simulink model "TNN_model"  (R2024b)
settings: Solver=VariableStepAuto  StartTime=0.0  StopTime=stopTime  RelTol=1e-3
values from neighbouring files (symbols this model uses):
  initialCondition = squeeze(test_tensor(numInputs+1:end,:,1))    [TNN_matlab.m]
  modelParams = exportToSimulink(model)    [TNN_matlab.m]
  testID = 1    [TNN_matlab.m]
undefined symbols (not defined in the file or in its folder): extractdata
settings Model: Creator=cstockha  LastModifiedBy=cstockha
settings DebuggingCC: UnderspecifiedInitializationDetection=Classic  MergeDetectMultiDrivingBlocksExec=none
settings ModelReferenceCC: PropagateSignalLabelsOutOfModel=off

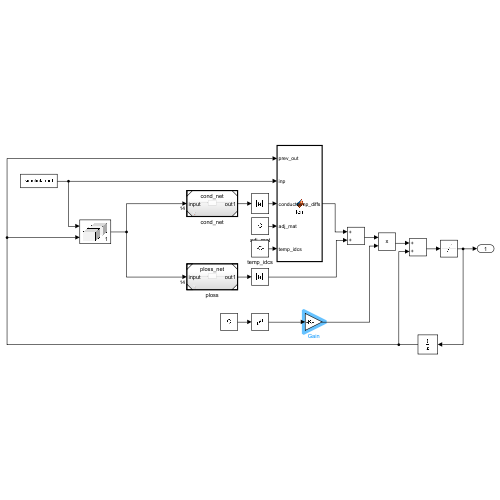
[thumbnail: Simulink's stored preview of the top-level diagram]
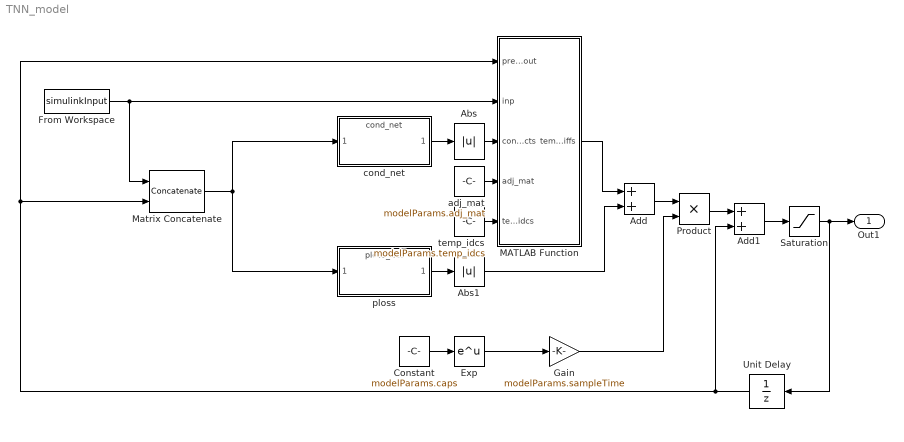
== system TNN_model ==
  Abs : Abs  SaturateOnIntegerOverflow=off
  Abs1 : Abs  SaturateOnIntegerOverflow=off
  Add : Sum  OutDataTypeStr=single
  Add1 : Sum
  Constant : Constant  Value=modelParams.caps
  Exp : Math
  From Workspace : FromWorkspace  VariableName=simulinkInput  SampleTime=1
  Gain : Gain  Gain=modelParams.sampleTime
  MATLAB Function : MATLAB Function  TreatAsAtomicUnit=on
  Matrix Concatenate : Concatenate  Mode=Multidimensional array
  Product : Product
  Saturation : Saturate  UpperLimit=5  LowerLimit=-1
  Unit Delay : UnitDelay  InitialCondition=extractdata(initialCondition(:,testID))  SampleTime=-1  HasFrameUpgradeWarning=on
  adj_mat : Constant  Value=modelParams.adj_mat
  cond_net : ModelReference  ModelNameDialog=cond_net  SimulationMode=Normal  ModelReferenceVersion=1.1
  ploss : ModelReference  ModelNameDialog=ploss_net  SimulationMode=Normal  ModelReferenceVersion=1.1
  temp_idcs : Constant  Value=modelParams.temp_idcs  VectorParams1D=off
  Out1 : Outport
  wires:
  cond_net/1 -> Abs/1
  ploss/1 -> Abs1/1
  Saturation/1 -> Out1/1, Unit Delay/1
  adj_mat/1 -> MATLAB Function/4(adj_mat)
  Add/1 -> Product/1
  temp_idcs/1 -> MATLAB Function/5(temp_idcs)
  Abs/1 -> MATLAB Function/3(conducts)
  MATLAB Function/1(temp_diffs) -> Add/1
  Abs1/1 -> Add/2
  Unit Delay/1 -> Matrix Concatenate/2, MATLAB Function/1(prev_out), Add1/2
  From Workspace/1 -> MATLAB Function/2(inp), Matrix Concatenate/1
  Matrix Concatenate/1 -> cond_net/1, ploss/1
  Constant/1 -> Exp/1
  Product/1 -> Add1/1
  Exp/1 -> Gain/1
  Gain/1 -> Product/2
  Add1/1 -> Saturation/1

== matlab function TNN_model/MATLAB Function ==
  data: prev_out input; inp input; conducts input; temp_diffs output; adj_mat input; temp_idcs input
function temp_diffs = fcn(prev_out,inp,conducts, adj_mat, temp_idcs)
temps = [prev_out; inp(temp_idcs,1)]';
conductArray = conducts(adj_mat);
temp_diffs = sum((temps - prev_out) .* conductArray, 2);
end
